simulink model "fig5_5_simulink"  (R2021b)
settings: Solver=ode45  StartTime=0.0  StopTime=50  MaxStep=0.01  RelTol=1e-3  EnableMultiTasking=on
undefined symbols (not defined in the file or in its folder): gama
settings Model: Creator=Guest  LastModifiedBy=One Informatic
settings SolverCC: AlgebraicLoopSolver=TrustRegion
settings DataIOCC: LimitDataPoints=on  SaveFormat=Array  ReturnWorkspaceOutputs=off
settings OptimizationCC: LifeSpan=inf
settings DebuggingCC: UnderspecifiedInitializationDetection=Classic  MergeDetectMultiDrivingBlocksExec=none  SolverPrmCheckMsg=warning  StateNameClashWarn=warning  SFUnexpectedBacktrackingDiag=warning  SFNoUnconditionalDefaultTransitionDiag=warning  SFExecutionAtInitializationDiag=none  SFMachineParentedDataDiag=warning  ArithmeticOperatorsInVariantConditions=warning
settings HardwareCC: ProdBitPerPointer=32  ProdBitPerSizeT=32  ProdBitPerPtrDiffT=32  ProdLargestAtomicFloat=None  ProdIntDivRoundTo=Undefined  ProdEndianess=Unspecified  ProdWordSize=32  ProdHWDeviceType=32-bit Generic
settings ModelReferenceCC: PropagateSignalLabelsOutOfModel=off
settings SFSimCC: SimUseLocalCustomCode=off  CustomCodeUndefinedFunction=UseInterfaceOnly
settings RTWCC: RTWUseLocalCustomCode=off
settings CodeAppCC: StateflowObjectComments=on
settings GRTTargetCC: TargetLangStandard=C89/C90 (ANSI)
settings ConfigComp: CovMetricSettings=dw  CovSaveCumulativeToWorkspaceVar=on  CovSaveSingleToWorkspaceVar=on  CovExternalEMLEnable=off

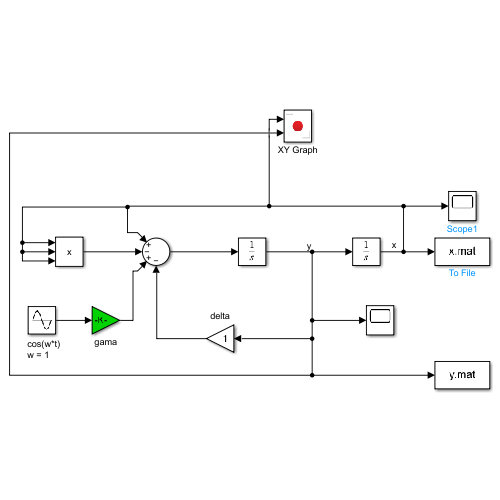
[thumbnail: Simulink's stored preview of the top-level diagram]
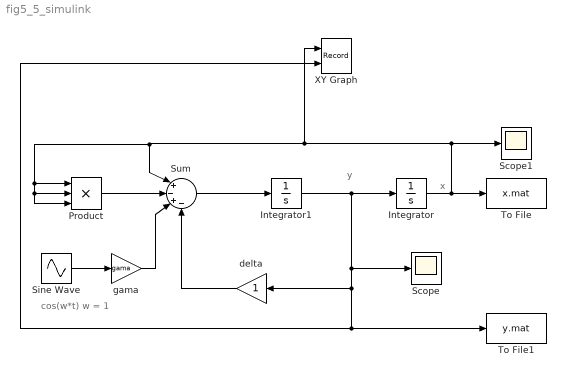
== system fig5_5_simulink ==
  note: y
  note: x
  note: cos(w*t)
      | w = 1
  Integrator : Integrator  InitialCondition=0.4
  Integrator1 : Integrator  InitialCondition=0.4
  Product : Product  Inputs=3
  Scope : Scope
  Scope1 : Scope
  Sine Wave : Sin  Phase=pi/2  SampleTime=0
  Sum : Sum  Inputs=|+-+-
  To File : ToFile  Filename=x.mat  MatrixName=x
  To File1 : ToFile  Filename=y.mat  MatrixName=y
  XY Graph : Record  FileSettingsInternal="{\"entries\":[{\"content\":{\"excelSettings\":{\"content\":{},\"type\":\"Streamout.ExcelSettings\"}},\"type\":\"Streamout.FileSettingStorage\",\"uuid\":\"174947f5-cead-4837-b813-202f870a3ebf\"}],\"packageUris\":[\"http://schema.mathworks.com/mf0/streamout_blocks/R2020a\"],\"version\":\"1.0\"}"  Layout=[1 1]  SignalsInternal="{\"entries\":[{\"content\":{\"signals\":[{\"content\":{\"blockPath\":[\"fig5_5_simulink/XY Graph\"],\"channel\":[],\"dimensions\":[1],\"domain\":\"fig5_5_simulink/XY Graph\",\"lineColor\":\"#edb120\",\"plots\":[],\"port\":1,\"sid\":[\"\"],\"signalID\":123,\"signalName\":\"Integrator\"},\"type\":\"RecordBlkView.Signal\",\"uuid\":\"46063df0-3239-4c14-ba44-69b37a26072b\"},{\"content\":{\"blockPath\":[\"fig5_5_simulink/XY Graph\"],\"channel\":[],\"dimensions\":[1],\"domain\":\"fig5_5_simulink/XY Graph\",\"lineColor\":\"#7e2f8e\",\"plots\":[],\"port\":2,\"sid\":[\"\"],\"signalID\":127,\"signalName\":\"Integrator1\"},\"type\":\"RecordBlkView.Signal\",\"uuid\":\"78bf77ec-1ff5-452f-b09e-33b1bed913e2\"}]},\"type\":\"RecordBlkView.InputSignals\",\"uuid\":\"0daa14da-4e67-4267-84b2-ef5315736216\"}],\"packageUris\":[\"http://schema.mathworks.com/mf0/streamout_blocks/R2020a\"],\"version\":\"1.0\"}"  VisualizationBindings="{\"xyplotplugin\":{\"info\":[{\"series\":[],\"subplotID\":1}]}}"  CompatibilityTag=XY  st=-1
  delta : Gain
  gama : Gain  Gain=gama
  wires:
  Sum/1 -> Integrator1/1
  Integrator/1 -> To File/1, XY Graph/1, Sum/1, Product/3, Product/2, Product/1, Scope1/1
  Product/1 -> Sum/2
  Sine Wave/1 -> gama/1
  gama/1 -> Sum/3
  Integrator1/1 -> To File1/1, XY Graph/2, delta/1, Scope/1, Integrator/1
  delta/1 -> Sum/4
